simulink model "InterfacciaSeriale232"  (Simulink 7.5)
settings: Solver=FixedStepDiscrete  StartTime=0.0  StopTime=inf  FixedStep=0.001  RelTol=1e-3
settings Model: Creator=m.satler  LastModifiedBy=amministratore
settings OptimizationCC: InitFltsAndDblsToZero=on
settings DebuggingCC: StrictBusMsg=Warning

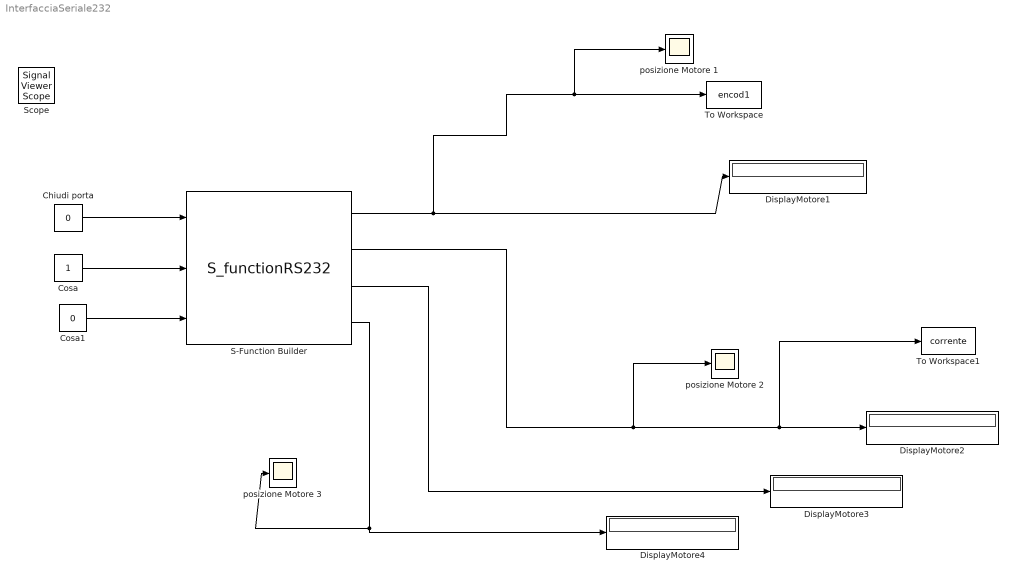
== system InterfacciaSeriale232 ==
  Chiudi porta : Constant  Value=0  OutDataTypeMode=int16  OutDataType=fixdt(1, 16)  OutScaling=2^0  OutDataTypeStr=int16
  Cosa : Constant  OutDataTypeMode=int8  OutDataType=fixdt(1, 16)  OutScaling=2^0  OutDataTypeStr=int8
  Cosa1 : Constant  Value=0  OutDataTypeMode=int8  OutDataType=fixdt(1, 16)  OutScaling=2^0  OutDataTypeStr=int8
  DisplayMotore{1..4} (4 alike) : Display
  S-Function Builder : S-Function  InitFcn=try, set_param(gcb,'FunctionName','S_functionRS232'), end  FunctionName=S_functionRS232  SFunctionModules=S_functionRS232_wrapper  WizardData=DataTag0  EnableBusSupport=off  mask(S-Function Builder){}
      mask help: The S-Function Builder block creates a wrapper C-MEX S-function from your supplied C code with multiple input ports, output ports, and a variable number of scalar, vector, or matrix parameters. The input and output ports can propagate Simulink built-in data types, fixed-point datatypes, complex, frame, 1-D, and 2-D signals. This block also supports discrete and continuous states of type real. You can optionally have the block generate a TLC file to be used with Real-Time Workshop for code generation.
      mask init:
      | val = [[.9  0.75 0.75 1 1 .9 .9 1]',[1 1 0.75 0.75 .9 .9 1 .9]'];try , sys = get_param(gcb,'SfunBuilderFcnName');if isempty(sys), sys = get_param(gcb,'FunctionName'); end,catch, sys = get_param(gcb,'FunctionName'); end
      settings: CopyFcn=set_param(gcbh,'LinkStatus','none')  PreSaveFcn=try, set_param(gcb,'FunctionName','S_functionRS232'), end  OpenFcn=sfunctionwizard(gcbh)
      mask Display:
      | plot(val(:,1),val(:,2)),disp(sys)
      | port_label('input',1,'Rif')
      | port_label('input',2,'chiudi')
      | port_label('input',3,'Switch')
      | port_label('output',1,'angle1')
      | port_label('output',2,'angle2')
      | port_label('output',3,'topolino')
      | port_label('output',4,'pippo')
  To Workspace : ToWorkspace  VariableName=encod1  SampleTime=-1  SaveFormat=Structure With Time
  To Workspace1 : ToWorkspace  VariableName=corrente  SampleTime=-1  SaveFormat=Structure With Time
  posizione Motore 1 : Scope
      settings: TimeRange=4.232356031954168  YMin=100.0841295595183  YMax=281.9722372453543
  posizione Motore 2 : Scope
      settings: TimeRange=10.64006650041563  YMin=-30000  YMax=30000
  posizione Motore 3 : Scope
      settings: TimeRange=10.64006650041563  YMin=-30000  YMax=30000  SaveName=ScopeData2
  Scope : SignalViewerScope  IOType=viewer  RefreshTime=0.035000
  wires:
  S-Function Builder/1 -> DisplayMotore1/1, To Workspace/1, posizione Motore 1/1
  Chiudi porta/1 -> S-Function Builder/1
  S-Function Builder/3 -> DisplayMotore3/1
  S-Function Builder/4 -> DisplayMotore4/1, posizione Motore 3/1
  S-Function Builder/2 -> DisplayMotore2/1, To Workspace1/1, posizione Motore 2/1
  Cosa1/1 -> S-Function Builder/3
  Cosa/1 -> S-Function Builder/2
